simulink model "uvms_sliding"  (Simulink 7.9)
settings: Solver=ode4  StartTime=0.0  StopTime=10.0  FixedStep=dt  RelTol=2*1e-3
values from neighbouring files (symbols this model uses):
  DH = struct('a',zeros(n,1),'d',zeros(n,1),'alpha',zeros(n,1))    [init.m]
  dt = 0.01    [run_simulation.m]
undefined symbols (not defined in the file or in its folder): commanded_zeta, ee_pose_init, Kinetics_Parameters, q_init, V_current, vehicle_euler_init, vehicle_position_init
(part 1 of 2)
settings Model: Creator=simena  LastModifiedBy=simena  SimulationMode=accelerator
settings OptimizationCC: SimCompilerOptimization=On
settings DebuggingCC: AlgebraicLoopMsg=error  UnderspecifiedInitializationDetection=Simplified
settings CodeAppCC: CustomSymbolStrType=$N$R$M_T

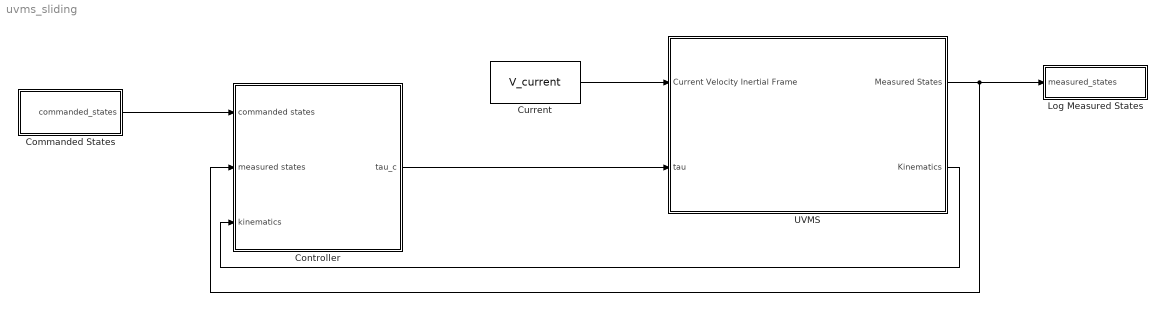
== system uvms_sliding ==
  Commanded States : Subsystem
  Controller : Subsystem
  Current : Constant  Value=V_current
  Log Measured States : Subsystem
  UVMS : Subsystem
  wires:
  Controller/1(tau_c) -> UVMS/2(tau)
  Commanded States/1(commanded_states) -> Controller/1(commanded states)
  UVMS/2(Kinematics) -> Controller/3(kinematics)
  UVMS/1(Measured States) -> Controller/2(measured states), Log Measured States/1(measured_states)
  Current/1 -> UVMS/1(Current Velocity Inertial Frame)

== system uvms_sliding/Commanded States ==
  To Workspace : ToWorkspace  VariableName=commanded_states_log  SampleTime=-1  SaveFormat=Timeseries
  commanded states : Subsystem  TreatAsAtomicUnit=on
  commanded_zeta : Constant  Value=commanded_zeta
  commanded_states : Outport
  wires:
  commanded_zeta/1 -> commanded states/1(zeta)
  commanded states/1(commanded_states) -> commanded_states/1, To Workspace/1

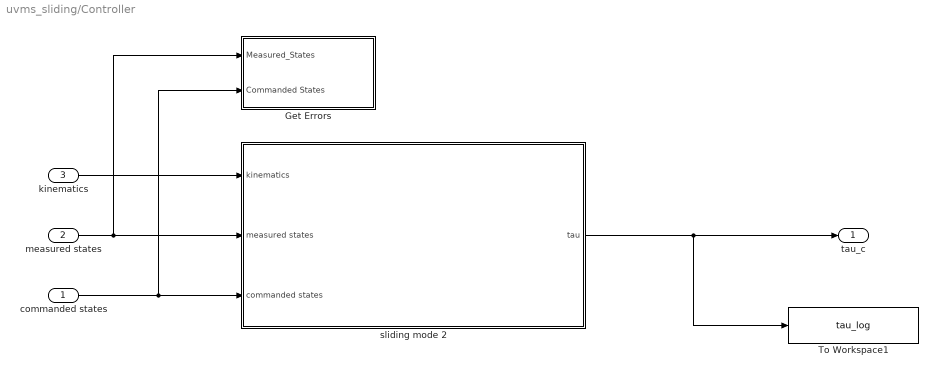
== system uvms_sliding/Controller ==
  commanded states : Inport
  measured states : Inport  Port=2
  kinematics : Inport  Port=3
  Get Errors : Subsystem
  To Workspace1 : ToWorkspace  VariableName=tau_log  SampleTime=-1  SaveFormat=Timeseries
  sliding mode 2 : Subsystem
  tau_c : Outport
  wires:
  kinematics/1 -> sliding mode 2/1(kinematics)
  measured states/1 -> sliding mode 2/2(measured states), Get Errors/1(Measured_States)
  commanded states/1 -> sliding mode 2/3(commanded states), Get Errors/2(Commanded States)
  sliding mode 2/1(tau) -> tau_c/1, To Workspace1/1

== system uvms_sliding/Log Measured States ==
  measured_states : Inport
  To Workspace1 : ToWorkspace  VariableName=measured_states_log  SampleTime=dt  SaveFormat=Timeseries
  wires:
  measured_states/1 -> To Workspace1/1

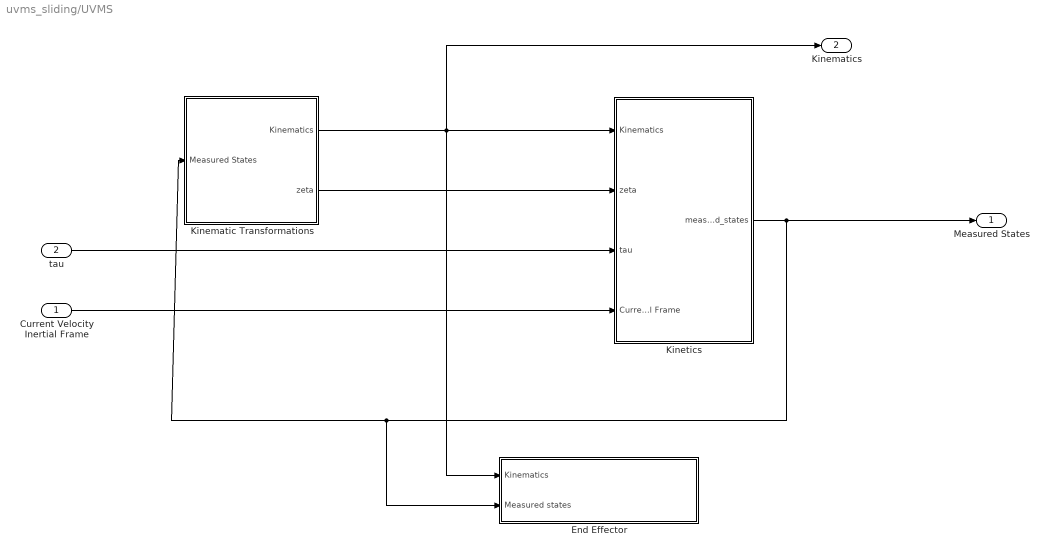
== system uvms_sliding/UVMS ==
  Current Velocity Inertial Frame : Inport
  tau : Inport  Port=2
  End Effector : Subsystem
  Kinematic Transformations : Subsystem  SystemSampleTime=dt
      settings: MinAlgLoopOccurrences=on
  Kinetics : Subsystem
      settings: MinAlgLoopOccurrences=on
  Measured States : Outport
  Kinematics : Outport  Port=2
  wires:
  Kinetics/1(measured_states) -> Kinematic Transformations/1(Measured States), End Effector/2(Measured states), Measured States/1
  Kinematic Transformations/1(Kinematics) -> Kinetics/1(Kinematics), End Effector/1(Kinematics), Kinematics/1
  Kinematic Transformations/2(zeta) -> Kinetics/2(zeta)
  tau/1 -> Kinetics/3(tau)
  Current Velocity Inertial Frame/1 -> Kinetics/4(Current Inertial Frame)

== system uvms_sliding/Commanded States/commanded states ==
  zeta : Inport
  Measure States : MATLAB Function  TreatAsAtomicUnit=on
  Reference system : Subsystem
  get dzeta : Subsystem
  zeta2xi : Subsystem
  commanded_states : Outport
  wires:
  Measure States/1(Commanded_States) -> commanded_states/1
  zeta2xi/1(xi) -> Measure States/3(xi)
  zeta/1 -> Reference system/1(In1)
  Reference system/1(Out1) -> Measure States/2(zeta), get dzeta/1(zeta), zeta2xi/1(zeta)
  get dzeta/1(dzeta) -> Measure States/1(dzeta)

== system uvms_sliding/Controller/Get Errors ==
  Measured_States : Inport
  Commanded States : Inport  Port=2
  Get error : MATLAB Function  TreatAsAtomicUnit=on
  Integrator : Integrator  InitialCondition=zeros(12,1)
  To Workspace : ToWorkspace  VariableName=error_states_log  SampleTime=-1  SaveFormat=Timeseries
  wires:
  Get error/2(Error_States) -> To Workspace/1
  Measured_States/1 -> Get error/1(Measured_States)
  Commanded States/1 -> Get error/2(Commanded_States)
  Integrator/1 -> Get error/3(integral_xi_tilde)
  Get error/1(integral_xi_tilde1) -> Integrator/1

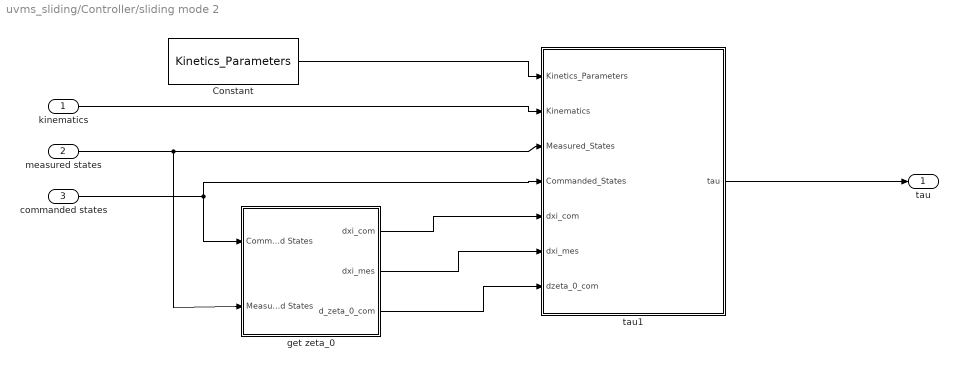
== system uvms_sliding/Controller/sliding mode 2 ==
  kinematics : Inport
  measured states : Inport  Port=2
  commanded states : Inport  Port=3
  Constant : Constant  Value=Kinetics_Parameters  OutDataTypeStr=Bus: kinetics_bus
  get zeta_0 : Subsystem
  tau1 : MATLAB Function  TreatAsAtomicUnit=on
  tau : Outport
  wires:
  Constant/1 -> tau1/1(Kinetics_Parameters)
  kinematics/1 -> tau1/2(Kinematics)
  measured states/1 -> tau1/3(Measured_States), get zeta_0/2(Measured States)
  tau1/1(tau) -> tau/1
  commanded states/1 -> tau1/4(Commanded_States), get zeta_0/1(Commanded States)
  get zeta_0/1(dxi_com) -> tau1/5(dxi_com)
  get zeta_0/2(dxi_mes) -> tau1/6(dxi_mes)
  get zeta_0/3(d_zeta_0_com) -> tau1/7(dzeta_0_com)

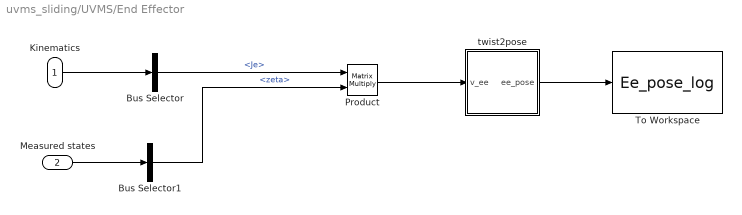
== system uvms_sliding/UVMS/End Effector ==
  Kinematics : Inport
  Measured states : Inport  Port=2
  Bus Selector : BusSelector  OutputSignals=Ji.Je
  Bus Selector1 : BusSelector  OutputSignals=zeta
  Product : Product  Multiplication=Matrix(*)  RndMeth=Zero
  To Workspace : ToWorkspace  VariableName=Ee_pose_log  SampleTime=dt  SaveFormat=Timeseries
  twist2pose : Subsystem
  wires:
  Product/1 -> twist2pose/1(v_ee)
  twist2pose/1(ee_pose) -> To Workspace/1
  Kinematics/1 -> Bus Selector/1
  Measured states/1 -> Bus Selector1/1
  Bus Selector/1 -> Product/1  "<Je>"
  Bus Selector1/1 -> Product/2  "<zeta>"

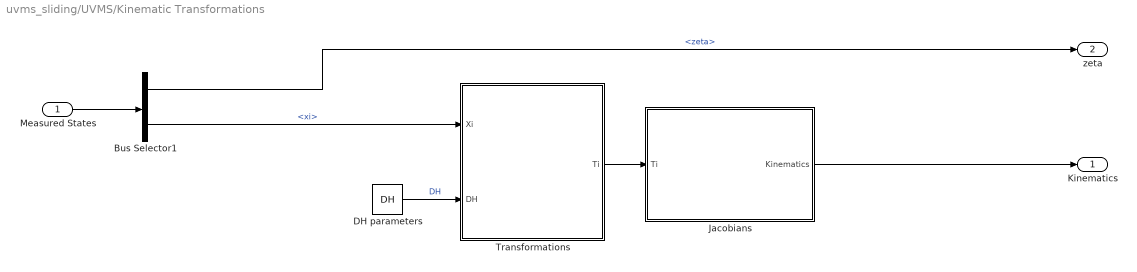
== system uvms_sliding/UVMS/Kinematic Transformations ==
  Measured States : Inport
  Bus Selector1 : BusSelector  OutputSignals=zeta,xi
  DH parameters : Constant  Value=DH  OutDataTypeStr=Bus: DH_bus
  Jacobians : MATLAB Function  TreatAsAtomicUnit=on  SystemSampleTime=dt
  Transformations : MATLAB Function  TreatAsAtomicUnit=on  SystemSampleTime=dt
  Kinematics : Outport
  zeta : Outport  Port=2
  wires:
  DH parameters/1 -> Transformations/2(DH)  "DH"
  Transformations/1(Ti) -> Jacobians/1(Ti)
  Bus Selector1/2 -> Transformations/1(Xi)  "<xi>"
  Bus Selector1/1 -> zeta/1  "<zeta>"
  Measured States/1 -> Bus Selector1/1
  Jacobians/1(Kinematics) -> Kinematics/1

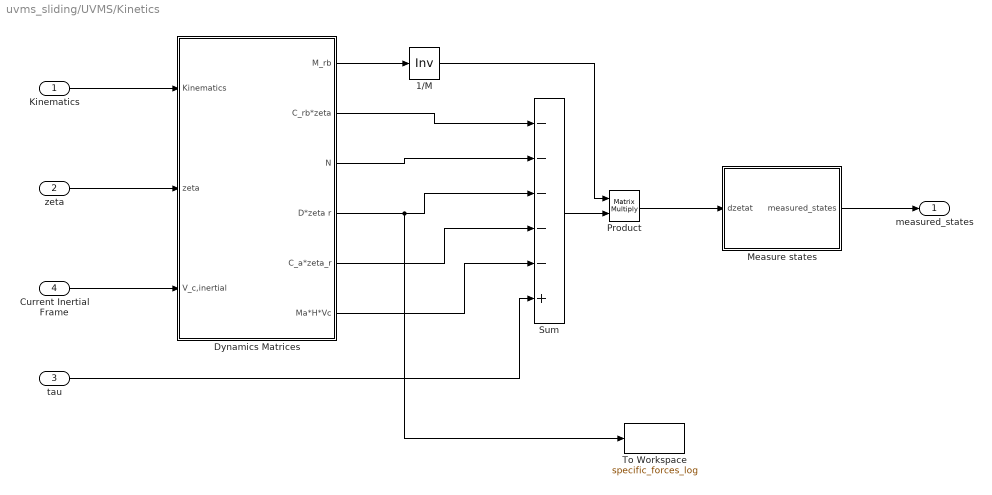
== system uvms_sliding/UVMS/Kinetics ==
  Kinematics : Inport
  zeta : Inport  Port=2
  tau : Inport  Port=3
  Current Inertial Frame : Inport  Port=4
  1/M : Product  Inputs=/  Multiplication=Matrix(*)
  Dynamics Matrices : Subsystem
  Measure states : Subsystem  TreatAsAtomicUnit=on
      settings: MinAlgLoopOccurrences=on
  Product : Product  Multiplication=Matrix(*)  RndMeth=Zero
  Sum : Sum  Inputs=-----+
  To Workspace : ToWorkspace  VariableName=specific_forces_log  SampleTime=-1  SaveFormat=Timeseries
  measured_states : Outport
  wires:
  Kinematics/1 -> Dynamics Matrices/1(Kinematics)
  Dynamics Matrices/1(M_rb) -> 1/M/1
  Sum/1 -> Product/2
  Product/1 -> Measure states/1(dzetat)
  Measure states/1(measured_states) -> measured_states/1
  1/M/1 -> Product/1
  Current Inertial Frame/1 -> Dynamics Matrices/3(V_c,inertial)
  zeta/1 -> Dynamics Matrices/2(zeta)
  Dynamics Matrices/2(C_rb*zeta) -> Sum/1
  Dynamics Matrices/3(N) -> Sum/2
  Dynamics Matrices/4(D*zeta r) -> Sum/3, To Workspace/1
  Dynamics Matrices/5(C_a*zeta_r) -> Sum/4
  Dynamics Matrices/6(Ma*H*Vc) -> Sum/5
  tau/1 -> Sum/6

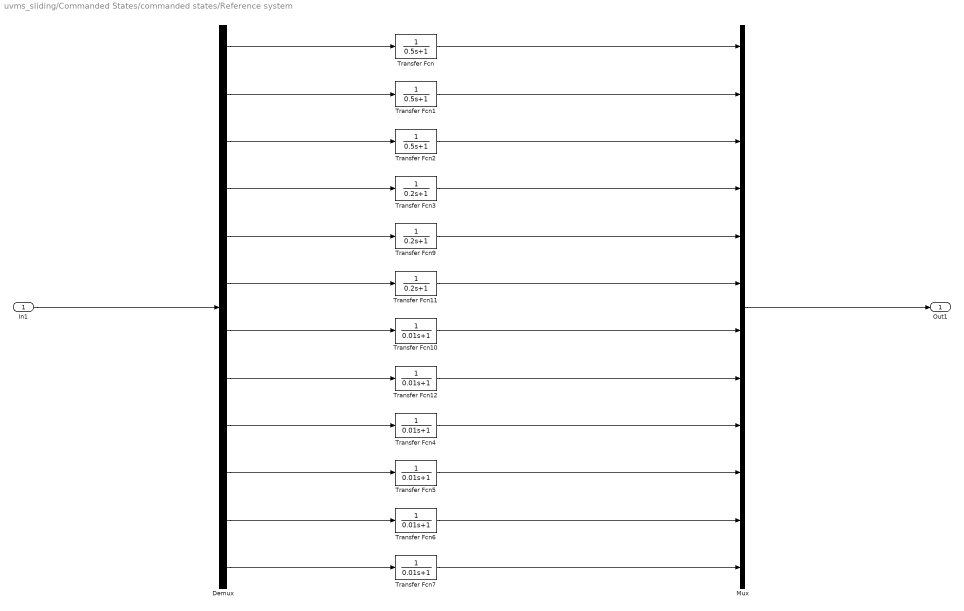
== system uvms_sliding/Commanded States/commanded states/Reference system ==
  In1 : Inport
  Demux : Demux  Outputs=12
  Mux : Mux  Inputs=12
  Transfer Fcn : TransferFcn  Denominator=[0.5 1]
  Transfer Fcn1 : TransferFcn  Denominator=[0.5 1]
  Transfer Fcn{4..7,10,12} (6 alike) : TransferFcn  Denominator=[0.01 1]
  Transfer Fcn11 : TransferFcn  Denominator=[0.2 1]
  Transfer Fcn2 : TransferFcn  Denominator=[0.5 1]
  Transfer Fcn3 : TransferFcn  Denominator=[0.2 1]
  Transfer Fcn9 : TransferFcn  Denominator=[0.2 1]
  Out1 : Outport
  wires:
  Demux/1 -> Transfer Fcn/1
  In1/1 -> Demux/1
  Transfer Fcn/1 -> Mux/1
  Demux/2 -> Transfer Fcn1/1
  Demux/3 -> Transfer Fcn2/1
  Demux/4 -> Transfer Fcn3/1
  Demux/5 -> Transfer Fcn9/1
  Demux/6 -> Transfer Fcn11/1
  Demux/7 -> Transfer Fcn10/1
  Demux/8 -> Transfer Fcn12/1
  Demux/9 -> Transfer Fcn4/1
  Demux/10 -> Transfer Fcn5/1
  Demux/11 -> Transfer Fcn6/1
  Demux/12 -> Transfer Fcn7/1
  Transfer Fcn1/1 -> Mux/2
  Transfer Fcn2/1 -> Mux/3
  Transfer Fcn3/1 -> Mux/4
  Transfer Fcn9/1 -> Mux/5
  Transfer Fcn11/1 -> Mux/6
  Transfer Fcn10/1 -> Mux/7
  Transfer Fcn12/1 -> Mux/8
  Transfer Fcn4/1 -> Mux/9
  Transfer Fcn5/1 -> Mux/10
  Transfer Fcn6/1 -> Mux/11
  Transfer Fcn7/1 -> Mux/12
  Mux/1 -> Out1/1

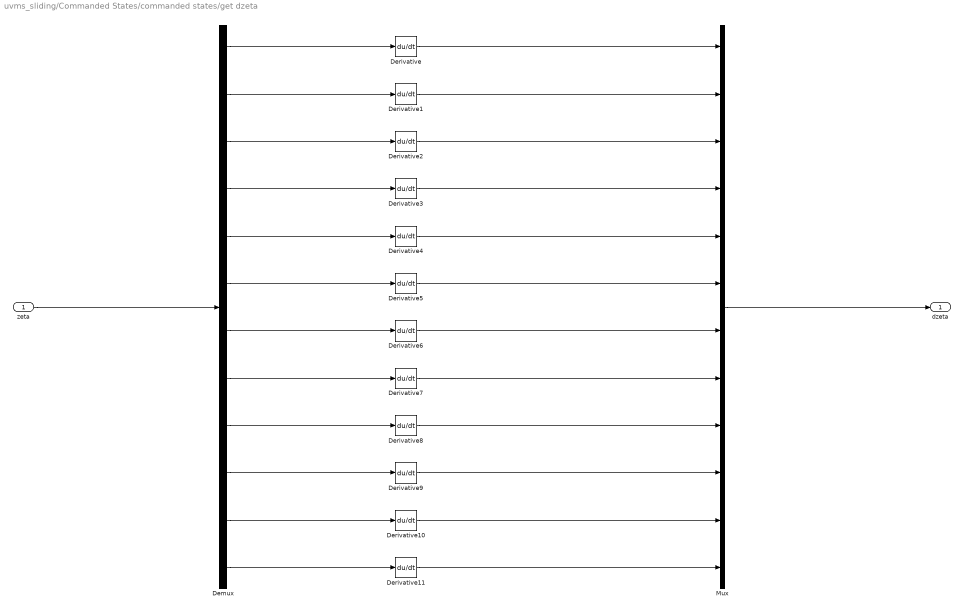
== system uvms_sliding/Commanded States/commanded states/get dzeta ==
  zeta : Inport
  Demux : Demux  Outputs=12
  Derivative{,1..11} (12 alike) : Derivative
  Mux : Mux  Inputs=12
  dzeta : Outport
  wires:
  Demux/1 -> Derivative/1
  zeta/1 -> Demux/1
  Derivative/1 -> Mux/1
  Demux/2 -> Derivative1/1
  Demux/3 -> Derivative2/1
  Demux/4 -> Derivative3/1
  Demux/5 -> Derivative4/1
  Demux/6 -> Derivative5/1
  Demux/7 -> Derivative6/1
  Demux/8 -> Derivative7/1
  Demux/9 -> Derivative8/1
  Demux/10 -> Derivative9/1
  Demux/11 -> Derivative10/1
  Demux/12 -> Derivative11/1
  Derivative1/1 -> Mux/2
  Derivative2/1 -> Mux/3
  Derivative3/1 -> Mux/4
  Derivative4/1 -> Mux/5
  Derivative5/1 -> Mux/6
  Derivative6/1 -> Mux/7
  Derivative7/1 -> Mux/8
  Derivative8/1 -> Mux/9
  Derivative9/1 -> Mux/10
  Derivative10/1 -> Mux/11
  Derivative11/1 -> Mux/12
  Mux/1 -> dzeta/1

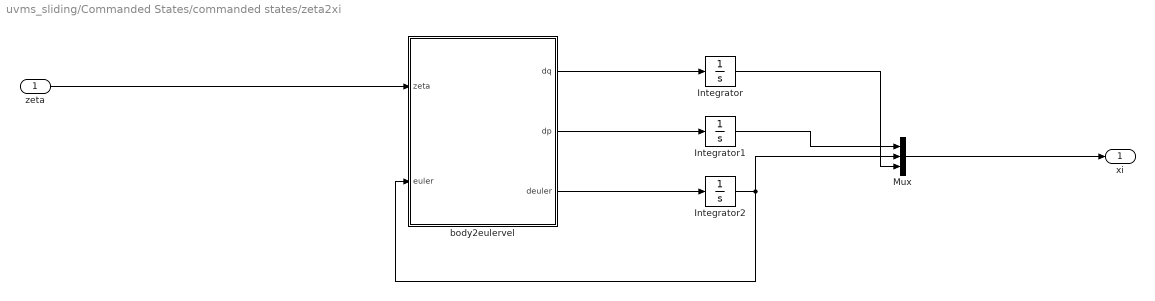
== system uvms_sliding/Commanded States/commanded states/zeta2xi ==
  zeta : Inport
  Integrator : Integrator  InitialCondition=q_init
  Integrator1 : Integrator  InitialCondition=vehicle_position_init
  Integrator2 : Integrator  InitialCondition=vehicle_euler_init
  Mux : Mux  Inputs=3
  body2eulervel : MATLAB Function  TreatAsAtomicUnit=on  SystemSampleTime=dt
  xi : Outport
  wires:
  body2eulervel/1(dq) -> Integrator/1
  body2eulervel/2(dp) -> Integrator1/1
  body2eulervel/3(deuler) -> Integrator2/1
  zeta/1 -> body2eulervel/1(zeta)
  Integrator2/1 -> body2eulervel/2(euler), Mux/2
  Mux/1 -> xi/1
  Integrator1/1 -> Mux/1
  Integrator/1 -> Mux/3

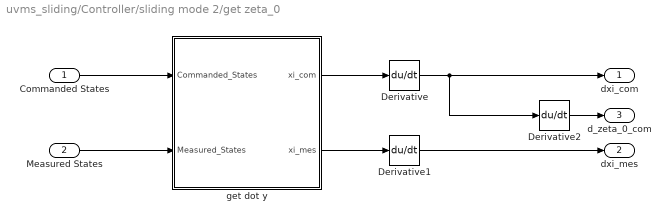
== system uvms_sliding/Controller/sliding mode 2/get zeta_0 ==
  Commanded States : Inport
  Measured States : Inport  Port=2
  Derivative : Derivative  CoefficientInTFapproximation=1000
  Derivative1 : Derivative  CoefficientInTFapproximation=1000
  Derivative2 : Derivative  CoefficientInTFapproximation=1000
  get dot y : MATLAB Function  TreatAsAtomicUnit=on
  dxi_com : Outport
  dxi_mes : Outport  Port=2
  d_zeta_0_com : Outport  Port=3
  wires:
  Commanded States/1 -> get dot y/1(Commanded_States)
  Measured States/1 -> get dot y/2(Measured_States)
  Derivative/1 -> dxi_com/1, Derivative2/1
  get dot y/1(xi_com) -> Derivative/1
  get dot y/2(xi_mes) -> Derivative1/1
  Derivative1/1 -> dxi_mes/1
  Derivative2/1 -> d_zeta_0_com/1

== system uvms_sliding/UVMS/End Effector/twist2pose ==
  v_ee : Inport
  Demux : Demux  Outputs=2
  Integrator : Integrator  InitialCondition=ee_pose_init
  Mux : Mux  Inputs=2
  body2eulervel : MATLAB Function  TreatAsAtomicUnit=on  SystemSampleTime=dt
  ee_pose : Outport
  wires:
  v_ee/1 -> body2eulervel/1(ee_velocity_twist)
  body2eulervel/1(ee_rates) -> Integrator/1
  Integrator/1 -> Demux/1
  Demux/2 -> body2eulervel/2(euler_angles_ee), Mux/2  "ee_angle"
  Demux/1 -> Mux/1  "ee_pos"
  Mux/1 -> ee_pose/1

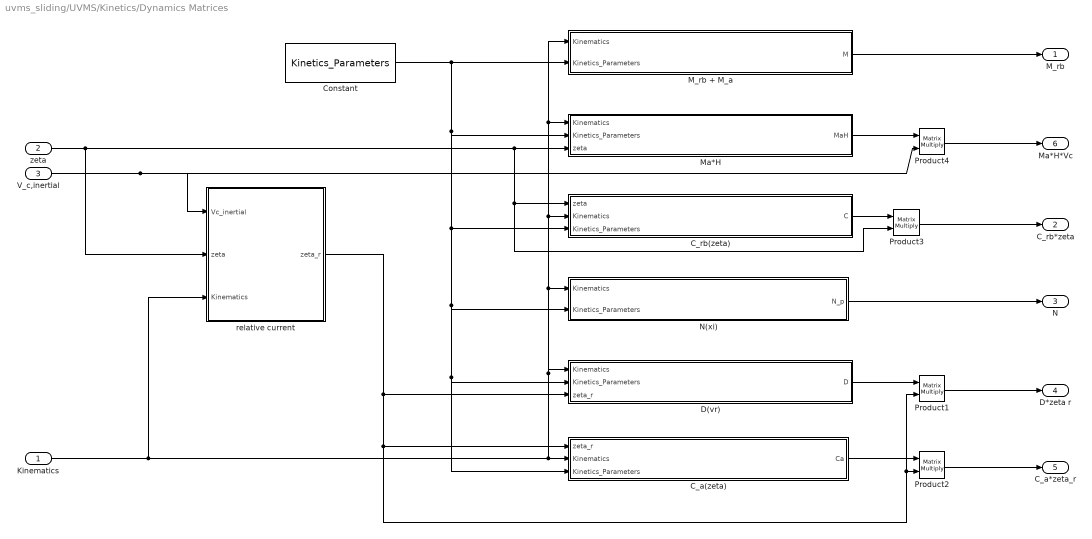
== system uvms_sliding/UVMS/Kinetics/Dynamics Matrices ==
  Kinematics : Inport
  zeta : Inport  Port=2
  V_c,inertial : Inport  Port=3
  C_a(zeta) : MATLAB Function  TreatAsAtomicUnit=on
  C_rb(zeta) : MATLAB Function  TreatAsAtomicUnit=on
  Constant : Constant  Value=Kinetics_Parameters  OutDataTypeStr=Bus: kinetics_bus
  D(vr) : MATLAB Function  TreatAsAtomicUnit=on
  M_rb + M_a : MATLAB Function  TreatAsAtomicUnit=on
  Ma*H : MATLAB Function  TreatAsAtomicUnit=on
  N(xi) : MATLAB Function  TreatAsAtomicUnit=on
  Product{1..4} (4 alike) : Product  Multiplication=Matrix(*)  RndMeth=Zero
  relative current : MATLAB Function  TreatAsAtomicUnit=on
  M_rb : Outport
  C_rb*zeta : Outport  Port=2
  N : Outport  Port=3
  D*zeta r : Outport  Port=4
  C_a*zeta_r : Outport  Port=5
  Ma*H*Vc : Outport  Port=6
  wires:
  Product1/1 -> D*zeta r/1
  Product2/1 -> C_a*zeta_r/1
  Product3/1 -> C_rb*zeta/1
  M_rb + M_a/1(M) -> M_rb/1
  Ma*H/1(MaH) -> Product4/1
  relative current/1(zeta_r) -> D(vr)/3(zeta_r), C_a(zeta)/1(zeta_r), Product2/2, Product1/2
  Kinematics/1 -> relative current/3(Kinematics), C_a(zeta)/2(Kinematics), D(vr)/1(Kinematics), N(xi)/1(Kinematics), C_rb(zeta)/2(Kinematics), Ma*H/1(Kinematics), M_rb + M_a/1(Kinematics)
  Constant/1 -> M_rb + M_a/2(Kinetics_Parameters), Ma*H/2(Kinetics_Parameters), C_rb(zeta)/3(Kinetics_Parameters), N(xi)/2(Kinetics_Parameters), C_a(zeta)/3(Kinetics_Parameters), D(vr)/2(Kinetics_Parameters)
  C_rb(zeta)/1(C) -> Product3/1
  N(xi)/1(N_p) -> N/1
  D(vr)/1(D) -> Product1/1
  C_a(zeta)/1(Ca) -> Product2/1
  zeta/1 -> Ma*H/3(zeta), Product3/2, C_rb(zeta)/1(zeta), relative current/2(zeta)
  V_c,inertial/1 -> Product4/2, relative current/1(Vc_inertial)
  Product4/1 -> Ma*H*Vc/1

== system uvms_sliding/UVMS/Kinetics/Measure states ==
  dzetat : Inport
  Integrator : Integrator
  Measure States : MATLAB Function  TreatAsAtomicUnit=on
  Unit Delay : UnitDelay  SampleTime=-1
  zeta2xi : Subsystem
  measured_states : Outport
  wires:
  dzetat/1 -> Integrator/1, Unit Delay/1
  Measure States/1(Measured_States) -> measured_states/1
  Integrator/1 -> Measure States/2(zeta), zeta2xi/1(zeta)
  zeta2xi/1(xi) -> Measure States/3(xi)
  Unit Delay/1 -> Measure States/1(dzeta)

== system uvms_sliding/UVMS/Kinetics/Measure states/zeta2xi ==
  zeta : Inport
  Integrator : Integrator  InitialCondition=q_init
  Integrator1 : Integrator  InitialCondition=vehicle_position_init
  Integrator2 : Integrator  InitialCondition=vehicle_euler_init
  Mux : Mux  Inputs=3
  body2eulervel : MATLAB Function  TreatAsAtomicUnit=on  SystemSampleTime=dt
  xi : Outport
  wires:
  body2eulervel/1(dq) -> Integrator/1
  body2eulervel/2(dp) -> Integrator1/1
  body2eulervel/3(deuler) -> Integrator2/1
  zeta/1 -> body2eulervel/1(zeta)
  Integrator2/1 -> body2eulervel/2(euler), Mux/2
  Mux/1 -> xi/1
  Integrator1/1 -> Mux/1
  Integrator/1 -> Mux/3

== matlab function UVMS/Kinematic Transformations/Jacobians ==
  data: Ti input Bus: Ti_bus; Kinematics output Bus: kin_bus
function Kinematics  = getJacobians(Ti)
%#codegen
    n=6;
    Ji = struct('Ji',zeros(n,n+6,n),'Je',zeros(n,n+6),'Jbe',zeros(n,n));
    Kinematics = struct('Ti', Ti, 'Ji',Ji);
    ji=zeros(6,6);
    for i=1:n
        ji=getji(Ti,i);
    
        Ji.Ji(:,:,i) = [Ti.Adgbi_inv(:,:,i), Ti.Adgbi_inv(:,:,i)*ji];
    end
    j6 = getje(Ti);
    Ji.Je = [Ti.Adgbe_inv, Ti.Adgbe_inv*j6];
    Ji.Jbe = Ti.Adgbe_inv*j6;
    Kinematics.Ji = Ji;
    Kinematics.Ti = Ti;
end




% return matrix Ji (see report)
function mat = getji(Ti,i)
    n=6;
    mat=zeros(6,6);
    Xii=[0,0,0,0,0,1]';
    mat(:,1)=eye(6)*Xii;
    for j=2:n
        if j<=i
            mat(:,j) = Ti.Adgbi(:,:,j-1)*Xii;
        end
    end

end

% return matrix Je (see report)
function mat = getje(Ti)
    n=6;
    mat=zeros(6,6);
    Xii=[0,0,0,0,0,1]';
    mat(:,1)=eye(6)*Xii;
    for i=2:(n-1)
        mat(:,i) = Ti.Adgbi(:,:,i-1)*Xii;
    end
    mat(:,6) = Ti.Adgbe*Xii;

end

function S = skew(v)
  S = [  0   -v(3)  v(2)
       v(3)  0    -v(1)
       -v(2) v(1)   0];
end

== matlab function UVMS/Kinematic Transformations/Transformations ==
  data: Xi input double; DH input Bus: DH_bus; Ti output Bus: Ti_bus
function Ti    = getTransformations(Xi,DH)
%#codegen
% Return transformations, rotations, positions and adjoint matrices for
% robot links
% Tbi.gbi(:,:,i) is the transformation from b to i etc
    n=6;    % number of links
    q=Xi(7:12);
    eta=Xi(1:6);
           
    Ti = struct('g0b',zeros(4,4),'g0i',zeros(4,4,n),'R0i', zeros(3,3,n),'R0b',zeros(3,3),'p0i', zeros(3,1,n), 'Adg0i',zeros(6,6,n),'Adg0i_inv',zeros(6,6,n),   ...
    'gbi',zeros(4,4,n),'Rbi', zeros(3,3,n),'pbi', zeros(3,1,n),'Adgbi',zeros(6,6,n),'Adgbi_inv',zeros(6,6,n),...
    'g6e',eye(4) ,'g0e',zeros(4,4),'R0e', zeros(3,3),'p0e', zeros(3,1),  'Adg0e',zeros(6,6),'Adg0e_inv',zeros(6,6),   ...
    'gbe',zeros(4,4),'Rbe', zeros(3,3),'pbe', zeros(3,1),'Adgbe',zeros(6,6),'Adgbe_inv',zeros(6,6) ...
    );
        
    Ti.g0b=eta2g0b(eta);
    Ti.R0b = Ti.g0b(1:3,1:3);

    % initial matrices 
    g=eye(4);
    g0=Ti.g0b;
    
    for i=1:n
       % transformations from frame b to frame i
       Ti.gbi(:,:,i) = g*getHom(q,DH,i);
       Ti.Rbi(:,:,i) = getRot(Ti.gbi(:,:,i));
       Ti.pbi(:,:,i) = getPos(Ti.gbi(:,:,i));
       Ti.Adgbi(:,:,i) = getAdgbi(Ti.Rbi(:,:,i), Ti.pbi(:,:,i) );
       Ti.Adgbi_inv(:,:,i) = getAdgbi_inv(Ti.Rbi(:,:,i), Ti.pbi(:,:,i) );
       g=Ti.gbi(:,:,i);
       % transformations from frame 0 to frame i
       Ti.g0i(:,:,i) = g0*getHom(q,DH,i);
       Ti.R0i(:,:,i) = getRot(Ti.g0i(:,:,i));
       Ti.p0i(:,:,i) = getPos(Ti.g0i(:,:,i));
       Ti.Adg0i(:,:,i) = getAdgbi(Ti.R0i(:,:,i), Ti.p0i(:,:,i) );
       Ti.Adg0i_inv(:,:,i) = getAdgbi_inv(Ti.R0i(:,:,i), Ti.p0i(:,:,i) );
       g0=Ti.g0i(:,:,i);
    end
    
    % transformation from frame 0 to ee
    g0e = Ti.g0i(:,:,6)*Ti.g6e;
    Ti.g0e = g0e;
    Ti.R0e = getRot(g0e);
    Ti.p0e = getPos(g0e);
    Ti.Adg0e = getAdgbi(Ti.R0e, Ti.p0e );
    Ti.Adg0e_inv = getAdgbi_inv(Ti.R0e, Ti.p0e);
        
    % transformation from frame b to ee
    gbe = Ti.gbi(:,:,6)*Ti.g6e;
    Ti.gbe = gbe;
    Ti.Rbe = getRot(gbe);
    Ti.pbe = getPos(gbe);
    Ti.Adgbe = getAdgbi(Ti.Rbe , Ti.pbe );
    Ti.Adgbe_inv = getAdgbi_inv(Ti.Rbe , Ti.pbe );
    
    % DEBUG
    coder.extrinsic('disp');
    coder.extrinsic('num2str');
    %if counter == 12        
%         disp(['------iteration: ' num2str(counter)]);
%         q';
%         [phi, theta,psi]=myR2euler(Ti.R0i(:,:,1))
%         Ti.g0i(:,:,1)
       %Ti.Adgbi(:,:,1)
       %Ti.Adgbi_inv(:,:,1)
       %Ti.pbi(:,1)
       %Ti.p0i(:,1)
       
    %end
    
 end




% homogenous transformation matrix - DH convention
% mat=Rot_z(theta)Trans_z(d)Trans_x(a)Rot_x(alpha)
function mat=getHom(q,DH,i)
    alpha=DH.alpha(i);
    a=DH.a(i);
    d=DH.d(i);
    theta=q(i);
    mat=eye(4);
    mat=[cos(theta), -sin(theta)*cos(alpha), sin(theta)*sin(alpha), a*cos(theta);
         sin(theta), cos(theta)*cos(alpha), -cos(theta)*sin(alpha), a*sin(theta);
         0, sin(alpha), cos(alpha), d;
         0,0,0,1
    ];

end

% extract position from homogenous 
% matrix
function vec = getPos(g)
    vec=g(1:3,4);
end

% extract rotation matrix-part out of
% homogenous matrix
function mat = getRot(g)
    mat=g(1:3,1:3);
end

function mat = getAdgbi(R,p)
    mat = zeros(6,6);
    ps=skew(p);
    mat=[R , ps*R ; zeros(3,3), R ];
end

function mat = getAdgbi_inv(R,p)
    mat = zeros(6,6);
    Rt=transpose(R);
    ps=skew(p);
    mat=[Rt , -Rt*ps ; zeros(3,3), Rt ];
end

function [phi,theta,psi] = myR2euler(R)
    phi   = atan2(R(3,2),R(3,3));
    theta = -asin(R(3,1));
    psi   = atan2(R(2,1),R(1,1));
end

function mat = eta2g0b(eta)
    mat = zeros(4,4);
    R=Rzyx(eta(4),eta(5),eta(6));
    pos=[eta(1); eta(2); eta(3)];
    mat = [R,pos;0,0,0,1];
end

function R = Rzyx(phi,theta,psi)
    cphi = cos(phi);
    sphi = sin(phi);
    cth  = cos(theta);
    sth  = sin(theta);
    cpsi = cos(psi);
    spsi = sin(psi);
    R = [...
       cpsi*cth  -spsi*cphi+cpsi*sth*sphi  spsi*sphi+cpsi*cphi*sth
       spsi*cth  cpsi*cphi+sphi*sth*spsi   -cpsi*sphi+sth*spsi*cphi
       -sth      cth*sphi                  cth*cphi ];
end

== matlab function UVMS/End Effector/twist2pose/body2eulervel ==
  data: ee_velocity_twist input double size=6; ee_rates output double size=6; euler_angles_ee input double size=3
function ee_rates = fcn(ee_velocity_twist, euler_angles_ee)                       
    %#codegen
       
    phi=euler_angles_ee(1);
    theta=euler_angles_ee(2);
    psi=euler_angles_ee(3);
    
    
    cphi = cos(phi);
    sphi = sin(phi);
    cth  = cos(theta);
    sth  = sin(theta);
 
    J1 = Rzyx(phi,theta,psi);
 
    if cth==0, error('J2 is singular for theta = +-90 degrees'); end
 
    J2 = [...
      1  sphi*sth/cth  cphi*sth/cth;
      0  cphi          -sphi;
      0  sphi/cth      cphi/cth ];
 
    J = [ J1  zeros(3,3);
      zeros(3,3) J2 ];
        
    ee_rates = zeros(6,1);
    ee_rates=J*ee_velocity_twist;
end



function R = Rzyx(phi,theta,psi)
    cphi = cos(phi);
    sphi = sin(phi);
    cth  = cos(theta);
    sth  = sin(theta);
    cpsi = cos(psi);
    spsi = sin(psi);

    R = [...
       cpsi*cth  -spsi*cphi+cpsi*sth*sphi  spsi*sphi+cpsi*cphi*sth
       spsi*cth  cpsi*cphi+sphi*sth*spsi   -cpsi*sphi+sth*spsi*cphi
       -sth      cth*sphi                  cth*cphi ];
end

== matlab function UVMS/Kinetics/Dynamics Matrices/M_rb + M_a ==
  data: Kinematics input Bus: kin_bus; M output double; Kinetics_Parameters input Bus: kinetics_bus
function M = getInertiaMatrix(Kinematics, Kinetics_Parameters)
%#codegen
%   getInertiaMatrix Returns the sum of the Rigid body inertia and the added mass:
%   M_rb + M_a
%   
    n=6;
    i=1;
    M = zeros(12,12);
    Inertia = Kinetics_Parameters.Inertia;
    AddedInertia = Kinetics_Parameters.AddedInertia;
    Jgb = [eye(6), zeros(6,6)];                                 % Jacobian from vehicle 
    Ji=Jgb;
    Hi = Kinetics_Parameters.Persistent.Hrg(:,:,i);
    Ii=Hi'*(Inertia(:,:,1) + AddedInertia(:,:,1))*Hi;           % Inertia of vehicle in CO
    M=M+(Ji')*Ii*Ji;
    for i=1:n
        Ji = Kinematics.Ji.Ji(:,:,i);                           % body jacobian
        Hi =Kinetics_Parameters.Persistent.Hrg(:,:,i+1);        % get Transformation matrix of link i
        Ii=Hi'*(Inertia(:,:,i+1) + AddedInertia(:,:,i+1))*Hi;   % Transform Inertia matrix from CG to CO
        M=M+(Ji')*Ii*Ji;                                        % Add link i's inertia to total inertia
    end
end

== matlab function UVMS/Kinetics/Dynamics Matrices/C_rb(zeta) ==
  data: zeta input double size=12; C output double; Kinematics input Bus: kin_bus; Kinetics_Parameters input Bus: kinetics_bus
function C = Coriolis(zeta,Kinematics,Kinetics_Parameters)
%-----------------------------------------------------------------------
%#codegen
%
%   This function calculates the coriolis according to From and Pettersen
%   (2013).
%-----------------------------------------------------------------------
    n=6;
    C=zeros(12,12);
    Inertia=Kinetics_Parameters.Inertia;
    Jis = Kinematics.Ji.Ji;
    
    % i = b
    Jgb = [eye(6), zeros(6,6)];
    i=1;
    Hi = Kinetics_Parameters.Persistent.Hrg(:,:,i);
    Ii=Hi'*Inertia(:,:,i);
    Wb = getWb(Ii,zeta);
    C = - (Jgb')*Wb*Hi*Jgb;     % time derivative of Jgb = 0  
    
    % i >=1
    for i=1:n
        Hi = Kinetics_Parameters.Persistent.Hrg(:,:,i+1);
        Ii=Hi'*Inertia(:,:,i+1);
        Wi=getWi(Ii,Jis(:,:,i), zeta);
        Jgi_dot=getJgi_dot(Kinematics, zeta,i);
        Jgi = Jis(:,:,i);
        
        C = C + (Jgi')*Ii*Hi*Jgi_dot - (Jgi')*Wi*Hi*Jgi;
    end
end



function Wb = getWb(I , zeta)
% Get the matrix Wi for i=b
% I: Inertia matrix for vehicle
% zeta: generalized velocity
    Wb = zeros(6,6);
    v = zeta(1:3);
    omega = zeta(4:6);
    mI = I(1:3,1:3); % Identity matrix times mass of link b
    Ib = I(4:6,4:6); % Moment of inertia
    mrgb = I(4:6,1:3); % mass times skew symmetric r_g^b
    dKv= mI*v - mrgb*omega;
    dKomega = Ib*omega + mrgb*v;
    
    Wb = [zeros(3,3), skew(dKv) ; skew(dKv), skew(dKomega)];
end

function Wi = getWi(I, Ji,zeta)
% Get matrix Wi for robot links
% I: inertia matrix for link i
% Ji: Jacobian for link i
% zeta: generalized coordinates
    Wi = zeros(6,6);
    V0i = Ji*zeta;
    v = V0i(1:3);
    omega = V0i(4:6);
    mI = I(1:3,1:3); % Identity matrix times mass of link b
    Ib = I(4:6,4:6); % Moment of inertia
    mrgb = I(4:6,1:3); % mass times skew symmetric r_g^b
    dKv= mI*v - mrgb*omega;
    dKomega = Ib*omega + mrgb*v;
    Wi = [zeros(3,3), skew(dKv) ; skew(dKv), skew(dKomega)];
end

function Jgi_dot=getJgi_dot(Kinematics, zeta,i)
% the functions below is related to Jgi_dot
    Jgi_dot = zeros(6,6+6);
    n=6;
    Jgi = Kinematics.Ji.Ji(:,:,i);
    omega = Jgi*zeta;
    Rbi = Kinematics.Ti.Rbi(:,:,i);
    pbi = Kinematics.Ti.pbi(:,i);
    omegaib = getOmegaib(Kinematics,zeta,i);
    dpbi =  getDpbi(Kinematics,zeta,i);
        
    dAdg_inv = [(Rbi')*skew(omegaib) , -(Rbi')*skew(omegaib)*skew(pbi) + (Rbi')*skew(dpbi); ...
                zeros(3,3) , (Rbi')*skew(omegaib) ];
    dJi = zeros(6,6);
    omega0b = zeta(4:6);
    
    % get d/dt(Ji)
    Xii=[0,0,0,0,0,1]';
    for k=2:n
       if k<=i
            dpbk = getDpbi(Kinematics, zeta ,k-1);
            Rbk= Kinematics.Ti.Rbi(:,:,k-1);
            omega0k = [zeros(3,3) , eye(3)]*Kinematics.Ji.Ji(:,:,k-1)*zeta;
            omegabk = omega0k - (Rbk')*omega0b;
            dJi(:,k) = [zeros(3,3), skew(dpbk)*Rbk*skew(omegabk) ...
                ; zeros(3,3) , (Rbk')*skew(omegabk)]*Xii;
       end
    end
    Ji=getji(Kinematics.Ti, i);
    Adg_inv = Kinematics.Ti.Adgbi_inv(:,:,i);
    Jgi_dot = [dAdg_inv, dAdg_inv*Ji + Adg_inv*dJi ];
end

function omegaib = getOmegaib(Kinematics,zeta,i)
% returns angular rage of vehcile wrt frame i noted in vehicle frame
    omegaib = zeros(3,1);
    Rbi = Kinematics.Ti.Rbi(:,:,i);
    Jgi = Kinematics.Ji.Ji(:,:,i);
    omega0b = zeta(4:6);
    omegaib = omega0b - Rbi*[zeros(3,3), eye(3)]*Jgi*zeta;
end

function dpbi = getDpbi( Kinematics, zeta,iter)
% returns time derivative of position vector of from frame b to frame i
    dpbi = zeros(3,1);
    H = [eye(3), zeros(3,3)];
    Rbi=Kinematics.Ti.Rbi(:,:,iter);
    Adgbi_inv = Kinematics.Ti.Adgbi_inv(:,:,iter);
    Ji = getji(Kinematics.Ti,iter);
    qd=zeros(6,1);
    qd(:,:)=zeta(7:12);
    dpbi = Rbi*H*Adgbi_inv*Ji*qd;
end


function mat = getji(Ti,i)
% return matrix Ji (see report)
    n=6;
    mat=zeros(6,6);
    Xii=[0,0,0,0,0,1]';
    mat(:,1)=eye(6)*Xii;
    for j=2:n
        if j<=i
            mat(:,j) = Ti.Adgbi(:,:,j-1)*Xii;
        end
    end
end

function S = skew(v)
  S = [  0   -v(3)  v(2)
       v(3)  0    -v(1)
       -v(2) v(1)   0];
end

== matlab function UVMS/Kinetics/Dynamics Matrices/N(xi) ==
  data: Kinematics input Bus: kin_bus; N_p output double; Kinetics_Parameters input Bus: kinetics_bus
function N_p = Persistent_Forces(Kinematics,Kinetics_Parameters)
%#codegen
%   N_p - 12 x 1 vector of generalized forces
%   Persistent_Forces returns the generalized forces due to boyancy and 
%   gravity

    %% init
    n=6;
    N_p=zeros(12,1);
    Jgis = Kinematics.Ji.Ji;
    
    %%  vehicle
    F_bp = getFbp(Kinematics, Kinetics_Parameters,1);           % Get wrench from persistent forces in CO
    Jbb=([eye(6), zeros(6,6)]);                                 % Jacobian from b to b
    N_p = Jbb'*F_bp;                                            % Get contribution to total forces through Jbb
    
    %% robot links
    for i=1:n
        Jgi=Jgis(:,:,i);                                        % Jacobian from b to i
        F_ip = getFip(Kinematics,Kinetics_Parameters, i+1);     % Get wrench in CO
        N_p = N_p + (Jgi')*F_ip;                                % Map to generalized forces and add to total
    end
    N_p = - N_p;                                                % reverse the sign to comply with the sign convention
end
    
    
function F_ip = getFip(Kinematics,Kinetics_Parameters, i)
% function calculating wrench from persistent forces 
% i=b: vehicle
% i>=1: robot arms
    F_ip = zeros(6,1);
    mi = Kinetics_Parameters.Persistent.m(i);
    g = Kinetics_Parameters.Persistent.g;
    rho = Kinetics_Parameters.Persistent.rho;
    nabla = Kinetics_Parameters.Persistent.nabla(i);
    Ri0 = Kinematics.Ti.R0i(:,:,i-1)';
    Hrg = Kinetics_Parameters.Persistent.Hrg(:,:,i);  
    Hrb = Kinetics_Parameters.Persistent.Hrb(:,:,i);
    ez=[0;0;1];
    F_ip(:,:) = (Hrg')*[-mi*g*Ri0*ez ;0;0;0]  + (Hrb')*[rho*nabla*g*Ri0*ez ;0;0;0 ];
end


function F_bp = getFbp(Kinematics,Kinetics_Parameters, i)
% function calculating wrench from persistent forces 
% i=b: vehicle
% i>=1: robot arms
    F_bp = zeros(6,1);
    mi = Kinetics_Parameters.Persistent.m(i);
    g = Kinetics_Parameters.Persistent.g;
    Hrg = Kinetics_Parameters.Persistent.Hrg(:,:,i);  
    Hrb = Kinetics_Parameters.Persistent.Hrb(:,:,i);
    rho = Kinetics_Parameters.Persistent.rho;
    nabla = Kinetics_Parameters.Persistent.nabla(i);
    Ri0 = (Kinematics.Ti.R0b)';
    ez=[0;0;1];
    F_bp(:,:) = (Hrg')*[-mi*g*Ri0*ez ; 0;0;0]  + (Hrb')*[rho*nabla*g*Ri0*ez ; 0;0;0 ];
end



function [phi,theta,psi] = myR2euler(R)
    phi   = atan2(R(3,2),R(3,3));
    theta = -asin(R(3,1));
    psi   = atan2(R(2,1),R(1,1));
end

== matlab function UVMS/Kinetics/Dynamics Matrices/relative current ==
  data: Vc_inertial input double; zeta input double; Kinematics input Bus: kin_bus; zeta_r output double
function zeta_r  = getRealtiveCurrent(Vc_inertial,zeta,Kinematics)
%#codegen

    %% init
    R0b = Kinematics.Ti.R0b;
    omega_0b = zeta(4:6);
    vc = Vc_inertial(1:3);


    %% get zeta relative of the current
    VcB =  [R0b'*vc;zeros(3,1)];
    zeta_r = zeta - [VcB; zeros(6,1)];
end

== matlab function UVMS/Kinetics/Dynamics Matrices/D(vr) ==
  data: Kinematics input double; D output double; Kinetics_Parameters input double; zeta_r input double
function D = fcn(Kinematics, Kinetics_Parameters,zeta_r)
%#codegen
%
% Returns the D matrix in the dynamics equation. The total forces is based
% on mappin the forces in each frame to the total generalized forces
% through the jacoian: tau = J^T*F_i. The forces in frame i is calculated
% from the forces in CG to CO through the transformation matrix: F_co =
% Hrg^T*F_cg
%
    %% init
    n=6;
    D=zeros(12,12);                                      % init matrix size
    HydroDynamics = Kinetics_Parameters.HydroDynamics;   % Hydrodynamics parameters
    Jgis = Kinematics.Ji.Ji;                             % Jacobians
    Hrgs = Kinetics_Parameters.Persistent.Hrg;           % Transformation matrix
    
    
    %% vehicle
    i=1;
    Jbb=[eye(6), zeros(6)];                               % Jacobian from frame 0 to frame b
    Hrg = Hrgs(:,:,i);                                    % Transformation matrix
    Vcg = Hrg*Jbb*zeta_r;                                   % velocity in CG mapped from CO
    Dcg =  HydroDynamics.Linear(:,:,i) + ...
           HydroDynamics.Quadratic(:,:,i)*diag(abs(Vcg)); % Wrench in CG
    Di = Hrg'*Dcg;                                        % Wrench in CO mapped from CG    
    D = Jbb'*Di*Jbb;                                      % Add contribution to the total matrix mapped from frame i 
                                                          % to generalized coordinates                                   
    
    %% robot links
    for i=1:n
        Jgi = Jgis(:,:,i);                                % Jacobian from frame 0 to frame i 
        Hrg = Hrgs(:,:,i+1);                              % Transformation matrix
        Vcg = Hrg*Jgi*zeta_r;                               % velocity in CG
        Dcg = HydroDynamics.Linear(:,:,i+1)+... 
          HydroDynamics.Quadratic(:,:,i+1)*diag(abs(Vcg));% Wrench in CG   
        Di = Hrg'*Dcg;                                    % Wrench in CO    
        D = D + Jgi'*Di*Jgi;                              % Add frame i's contribution to D matrix    
    end

end

== matlab function UVMS/Kinetics/Measure states/Measure States ==
  data: dzeta input double; Measured_States output Bus: measured_states_bus; zeta input double; xi input double
function Measured_States = fcn(dzeta, zeta, xi)
%#codegen

Measured_States.dzeta = dzeta;
Measured_States.zeta = zeta;
Measured_States.xi = xi;

end

== matlab function UVMS/Kinetics/Dynamics Matrices/C_a(zeta) ==
  data: zeta_r input double size=12; Ca output double; Kinematics input Bus: kin_bus; Kinetics_Parameters input Bus: kinetics_bus
function Ca = AddedCoriolis(zeta_r,Kinematics,Kinetics_Parameters)
%#codegen ..............................................
%
%   This function calculates the added coriolis matrix
%.......................................................
    n=6;
    Ca=zeros(12,12);
    Inertia=Kinetics_Parameters.AddedInertia;
    Jis = Kinematics.Ji.Ji;
    
    % vehicle
    Jgb = [eye(6), zeros(6,6)];
    i=1;
    Hi = Kinetics_Parameters.Persistent.Hrg(:,:,i+1);
    Ii=Hi'*Inertia(:,:,i);
    Wb = getWb(Ii,zeta_r);
    Ca = - (Jgb')*Wb*Hi*Jgb;     % time derivative of Jgb = 0  
    
    % manipulator links
    for i=1:n
        Hi = Kinetics_Parameters.Persistent.Hrg(:,:,i+1);
        Ii=Hi'*Inertia(:,:,i+1);
        Wi=getWi(Ii,Jis(:,:,i), zeta_r);
        Jgi_dot=getJgi_dot(Kinematics, zeta_r,i);
        Jgi = Jis(:,:,i);
        Ca = Ca + (Jgi')*Ii*Hi*Jgi_dot - (Jgi')*Wi*Hi*Jgi;
    end
end



function Wb = getWb(I , zeta)
% Get the matrix Wi for i=b
% I: Inertia matrix for vehicle
% zeta: generalized velocity
    Wb = zeros(6,6);
    v = zeta(1:3);
    omega = zeta(4:6);
    mI = I(1:3,1:3); % Identity matrix times mass of link b
    Ib = I(4:6,4:6); % Moment of inertia
    mrgb = I(4:6,1:3); % mass times skew symmetric r_g^b
    dKv= mI*v - mrgb*omega;
    dKomega = Ib*omega + mrgb*v;
    
    Wb = [zeros(3,3), skew(dKv) ; skew(dKv), skew(dKomega)];
end

function Wi = getWi(I, Ji,zeta)
% Get matrix Wi for robot links
% I: inertia matrix for link i
% Ji: Jacobian for link i
% zeta: generalized coordinates
    Wi = zeros(6,6);
    V0i = Ji*zeta;
    v = V0i(1:3);
    omega = V0i(4:6);
    mI = I(1:3,1:3); % Identity matrix times mass of link b
    Ib = I(4:6,4:6); % Moment of inertia
    mrgb = I(4:6,1:3); % mass times skew symmetric r_g^b
    dKv= mI*v - mrgb*omega;
    dKomega = Ib*omega + mrgb*v;
    Wi = [zeros(3,3), skew(dKv) ; skew(dKv), skew(dKomega)];
end

function Jgi_dot=getJgi_dot(Kinematics, zeta,i)
% the functions below is related to Jgi_dot
    Jgi_dot = zeros(6,6+6);
    n=6;
    Jgi = Kinematics.Ji.Ji(:,:,i);
    omega = Jgi*zeta;
    Rbi = Kinematics.Ti.Rbi(:,:,i);
    pbi = Kinematics.Ti.pbi(:,i);
    omegaib = getOmegaib(Kinematics,zeta,i);
    dpbi =  getDpbi(Kinematics,zeta,i);
        
    dAdg_inv = [(Rbi')*skew(omegaib) , -(Rbi')*skew(omegaib)*skew(pbi) + (Rbi')*skew(dpbi); ...
                zeros(3,3) , (Rbi')*skew(omegaib) ];
    dJi = zeros(6,6);
    omega0b = zeta(4:6);
    
    % get d/dt(Ji)
    Xii=[0,0,0,0,0,1]';
    for k=2:n
       if k<=i
            dpbk = getDpbi(Kinematics, zeta ,k-1);
            Rbk= Kinematics.Ti.Rbi(:,:,k-1);
            omega0k = [zeros(3,3) , eye(3)]*Kinematics.Ji.Ji(:,:,k-1)*zeta;
            omegabk = omega0k - (Rbk')*omega0b;
            dJi(:,k) = [zeros(3,3), skew(dpbk)*Rbk*skew(omegabk) ...
                ; zeros(3,3) , (Rbk')*skew(omegabk)]*Xii;
       end
    end
    Ji=getji(Kinematics.Ti, i);
    Adg_inv = Kinematics.Ti.Adgbi_inv(:,:,i);
    Jgi_dot = [dAdg_inv, dAdg_inv*Ji + Adg_inv*dJi ];
end

function omegaib = getOmegaib(Kinematics,zeta,i)
% returns angular rage of vehcile wrt frame i noted in vehicle frame
    omegaib = zeros(3,1);
    Rbi = Kinematics.Ti.Rbi(:,:,i);
    Jgi = Kinematics.Ji.Ji(:,:,i);
    omega0b = zeta(4:6);
    omegaib = omega0b - Rbi*[zeros(3,3), eye(3)]*Jgi*zeta;
end

function dpbi = getDpbi( Kinematics, zeta,iter)
% returns time derivative of position vector of from frame b to frame i
    dpbi = zeros(3,1);
    H = [eye(3), zeros(3,3)];
    Rbi=Kinematics.Ti.Rbi(:,:,iter);
    Adgbi_inv = Kinematics.Ti.Adgbi_inv(:,:,iter);
    Ji = getji(Kinematics.Ti,iter);
    qd=zeros(6,1);
    qd(:,:)=zeta(7:12);
    dpbi = Rbi*H*Adgbi_inv*Ji*qd;
end


function mat = getji(Ti,i)
% return matrix Ji (see report)
    n=6;
    mat=zeros(6,6);
    Xii=[0,0,0,0,0,1]';
    mat(:,1)=eye(6)*Xii;
    for j=2:n
        if j<=i
            mat(:,j) = Ti.Adgbi(:,:,j-1)*Xii;
        end
    end
end


function S = skew(v)
  S = [  0   -v(3)  v(2)
       v(3)  0    -v(1)
       -v(2) v(1)   0];
end

== matlab function UVMS/Kinetics/Measure states/zeta2xi/body2eulervel ==
  data: zeta input double size=12; dq output double size=6; dp output double; deuler output double size=3; euler input double
function [dq, dp, deuler] = fcn(zeta, euler)                       
    %#codegen
       
    phi=euler(1);
    theta=euler(2);
    psi=euler(3);
    
    
    cphi = cos(phi);
    sphi = sin(phi);
    cth  = cos(theta);
    sth  = sin(theta);
 
    J1 = Rzyx(phi,theta,psi);
 
    if cth==0, error('J2 is singular for theta = +-90 degrees'); end
 
    J2 = [...
      1  sphi*sth/cth  cphi*sth/cth;
      0  cphi          -sphi;
      0  sphi/cth      cphi/cth ];
 
    J = [ J1  zeros(3,3);
      zeros(3,3) J2 ];
        
    vehicle_velocity_twist = zeta(1:6);

    vehicle_rates=J*vehicle_velocity_twist;
    dp = vehicle_rates(1:3);
    deuler = vehicle_rates(4:6);
    dq = zeta(7:12);
end



function R = Rzyx(phi,theta,psi)
    cphi = cos(phi);
    sphi = sin(phi);
    cth  = cos(theta);
    sth  = sin(theta);
    cpsi = cos(psi);
    spsi = sin(psi);

    R = [...
       cpsi*cth  -spsi*cphi+cpsi*sth*sphi  spsi*sphi+cpsi*cphi*sth
       spsi*cth  cpsi*cphi+sphi*sth*spsi   -cpsi*sphi+sth*spsi*cphi
       -sth      cth*sphi                  cth*cphi ];
end

== matlab function UVMS/Kinetics/Dynamics Matrices/Ma*H ==
  data: Kinematics input double; Kinetics_Parameters input double; MaH output double; zeta input double
function MaH = fcn(Kinematics,Kinetics_Parameters,zeta)
%#codegen ..........................
%
%  returns rest of the the added mass
%  force matrix:
%       Ma*H(xi,zeta)
% ..................................
    n=6;
    i=1;
    
    %% get the total Added mass matrix
    Ma = zeros(12,12);
    AddedInertia = Kinetics_Parameters.AddedInertia;
    Jgb = [eye(6), zeros(6,6)];                                 % Jacobian from vehicle 
    Ji=Jgb;
    Hi = Kinetics_Parameters.Persistent.Hrg(:,:,i);
    Ii=Hi'*( AddedInertia(:,:,1))*Hi;                           % Inertia of vehicle in CO
    Ma=Ma+(Ji')*Ii*Ji;
    for i=1:n
        Ji = Kinematics.Ji.Ji(:,:,i);                           % body jacobian
        Hi =Kinetics_Parameters.Persistent.Hrg(:,:,i+1);        % get Transformation matrix of link i
        Ii=Hi'*(AddedInertia(:,:,i+1))*Hi;                      % Transform Inertia matrix from CG to CO
        Ma=Ma+(Ji')*Ii*Ji;                                      % Add link i's inertia to total inertia
    end
    
    %% calculate the matrix product
    H = zeros(12,6);
    R0b = Kinematics.Ti.R0b;
    omega0b = zeta(4:6);
    H(1:3,1:3) = R0b'*skew(omega0b);
    MaH = Ma*H;
end

function S = skew(v)
  S = [  0   -v(3)  v(2)
       v(3)  0    -v(1)
       -v(2) v(1)   0];
end

== matlab function Commanded States/commanded states/Measure States ==
  data: dzeta input double; Commanded_States output Bus: commanded_states_bus; zeta input double; xi input double
function Commanded_States = fcn(dzeta, zeta, xi)
%#codegen

Commanded_States.dzeta = dzeta;
Commanded_States.zeta = zeta;
Commanded_States.xi = xi;

end

== matlab function Commanded States/commanded states/zeta2xi/body2eulervel ==
  data: zeta input double size=12; dq output double size=6; dp output double; deuler output double size=3; euler input double
function [dq, dp, deuler] = fcn(zeta, euler)                       
    %#codegen
       
    phi=euler(1);
    theta=euler(2);
    psi=euler(3);
    
    
    cphi = cos(phi);
    sphi = sin(phi);
    cth  = cos(theta);
    sth  = sin(theta);
 
    J1 = Rzyx(phi,theta,psi);
 
    if cth==0, error('J2 is singular for theta = +-90 degrees'); end
 
    J2 = [...
      1  sphi*sth/cth  cphi*sth/cth;
      0  cphi          -sphi;
      0  sphi/cth      cphi/cth ];
 
    J = [ J1  zeros(3,3);
      zeros(3,3) J2 ];
        
    vehicle_velocity_twist = zeta(1:6);

    vehicle_rates=J*vehicle_velocity_twist;
    dp = vehicle_rates(1:3);
    deuler = vehicle_rates(4:6);
    dq = zeta(7:12);
end



function R = Rzyx(phi,theta,psi)
    cphi = cos(phi);
    sphi = sin(phi);
    cth  = cos(theta);
    sth  = sin(theta);
    cpsi = cos(psi);
    spsi = sin(psi);

    R = [...
       cpsi*cth  -spsi*cphi+cpsi*sth*sphi  spsi*sphi+cpsi*cphi*sth
       spsi*cth  cpsi*cphi+sphi*sth*spsi   -cpsi*sphi+sth*spsi*cphi
       -sth      cth*sphi                  cth*cphi ];
end

== matlab function Controller/Get Errors/Get error ==
  data: integral_xi_tilde1 output double; Measured_States input Bus: measured_states_bus; Commanded_States input Bus: commanded_states_bus; Error_States output Bus: error_states_bus; integral_xi_tilde input double
function [integral_xi_tilde1, Error_States] = fcn(Measured_States, Commanded_States, integral_xi_tilde)
%#codegen
    xi_tilde = Commanded_States.xi - Measured_States.xi  ;
    zeta_tilde = Commanded_States.zeta - Measured_States.zeta ;
    integral_xi_tilde1 = integral_xi_tilde;
    Error_States.dzeta_tilde = zeros(12,1);
    Error_States.zeta_tilde = zeta_tilde;
    Error_States.xi_tilde = xi_tilde;
    Error_States.integral_xi_tilde = integral_xi_tilde;
end

== matlab function Controller/sliding mode 2/get zeta_0/get dot y ==
  data: Commanded_States input double; xi_com output double; Measured_States input double; xi_mes output double
function [xi_com, xi_mes] = fcn(Commanded_States, Measured_States)
%#codegen
   xi_com = Commanded_States.xi;
   xi_mes = Measured_States.xi;
end
